simulink model "Filter_referencemodel"  (R2020a)
settings: Solver=FixedStepAuto  StartTime=0.0  StopTime=10.0  FixedStep=0.1  RelTol=1e-3
settings Model: Creator=Hp  LastModifiedBy=Hp
settings DataIOCC: SaveOutput=off  SaveTime=off

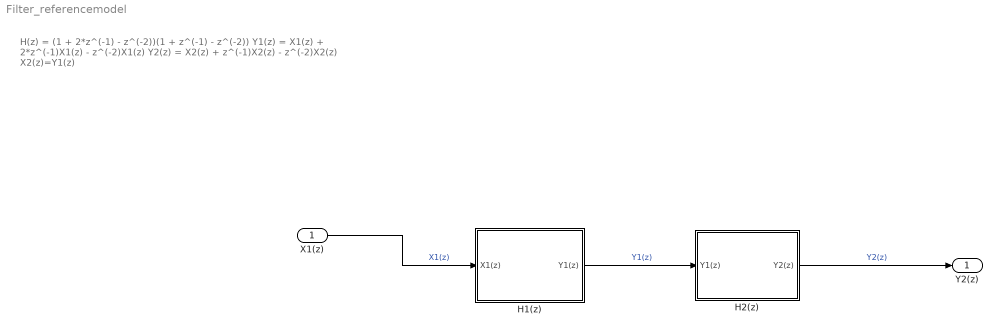
== system Filter_referencemodel ==
  note: H(z) = (1 + 2*z^(-1) - z^(-2))(1 + z^(-1) - z^(-2))
      |
      | Y1(z) = X1(z) + 2*z^(-1)X1(z) - z^(-2)X1(z)
      | Y2(z) = X2(z) + z^(-1)X2(z) - z^(-2)X2(z)
      | X2(z)=Y1(z)
  X1(z) : Inport  OutDataTypeStr=double  PortDimensions=1  SampleTime=[0.10000000000000001,0]
  H1(z) : Subsystem
  H2(z) : Subsystem
  Y2(z) : Outport  OutDataTypeStr=double  PortDimensions=1  SampleTime=[0.10000000000000001,0]
  wires:
  H1(z)/1(Y1(z)) -> H2(z)/1(Y1(z))  "Y1(z)"
  X1(z)/1 -> H1(z)/1(X1(z))  "X1(z)"
  H2(z)/1(Y2(z)) -> Y2(z)/1  "Y2(z)"

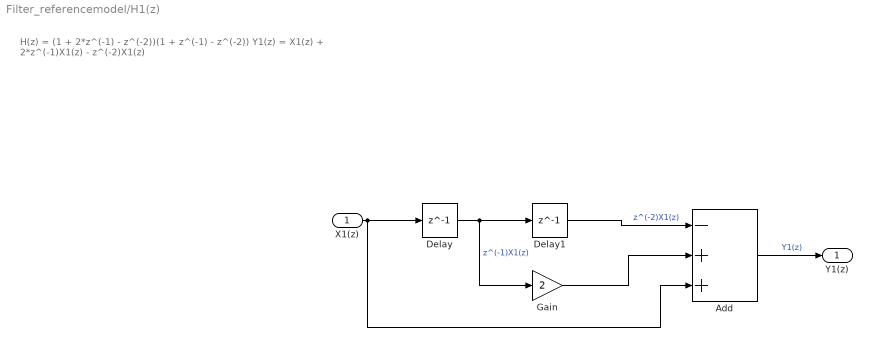
== system Filter_referencemodel/H1(z) ==
  note: H(z) = (1 + 2*z^(-1) - z^(-2))(1 + z^(-1) - z^(-2))
      |
      | Y1(z) = X1(z) + 2*z^(-1)X1(z) - z^(-2)X1(z)
  X1(z) : Inport
  Add : Sum  Inputs=-++
  Delay : Delay  DelayLength=1
  Delay1 : Delay  DelayLength=1
  Gain : Gain  Gain=2
  Y1(z) : Outport
  wires:
  X1(z)/1 -> Delay/1, Add/3
  Gain/1 -> Add/2
  Add/1 -> Y1(z)/1  "Y1(z)"
  Delay/1 -> Delay1/1, Gain/1  "z^(-1)X1(z)"
  Delay1/1 -> Add/1  "z^(-2)X1(z)"

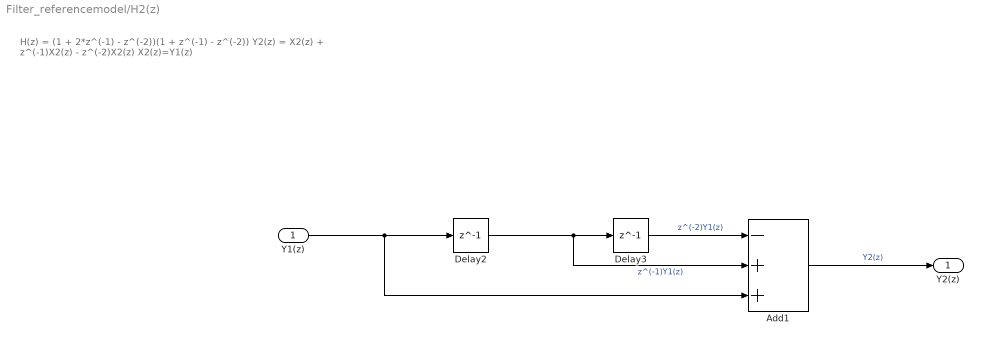
== system Filter_referencemodel/H2(z) ==
  note: H(z) = (1 + 2*z^(-1) - z^(-2))(1 + z^(-1) - z^(-2))
      |
      | Y2(z) = X2(z) + z^(-1)X2(z) - z^(-2)X2(z)
      | X2(z)=Y1(z)
  Y1(z) : Inport
  Add1 : Sum  Inputs=-++
  Delay2 : Delay  DelayLength=1
  Delay3 : Delay  DelayLength=1
  Y2(z) : Outport
  wires:
  Add1/1 -> Y2(z)/1  "Y2(z)"
  Delay3/1 -> Add1/1  "z^(-2)Y1(z)"
  Y1(z)/1 -> Delay2/1, Add1/3
  Delay2/1 -> Delay3/1, Add1/2  "z^(-1)Y1(z)"
